simulink subsystem "SimscapePWMModule"  (R2022b)
settings: Solver=VariableStepAuto  StartTime=0.0  StopTime=10.0  RelTol=1e-3
undefined symbols (not defined in the file): DeadTime, fsw
libraries: fl_lib x25
settings Model: Creator=ykamatan  LastModifiedBy=ykamatan

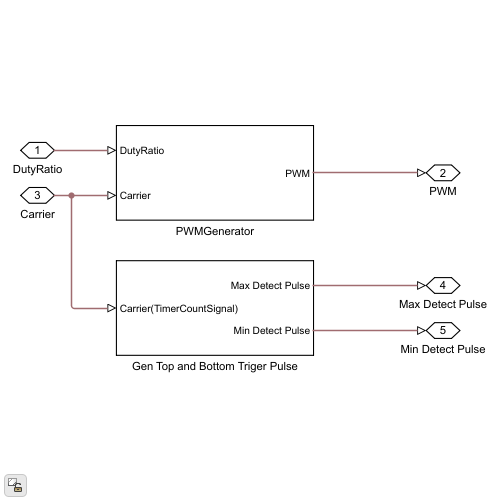
[thumbnail: Simulink's stored preview of the top-level diagram]
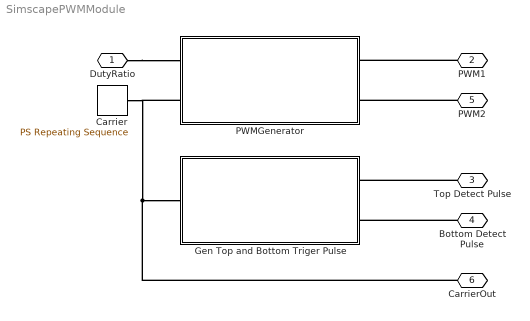
== system SimscapePWMModule ==
  Carrier : fl_lib/Physical Signals/Sources/PS Repeating Sequence  y_init=1  offset=0 s  sig_type=1  durations=[1/fsw/2 1/fsw/2] s  y_start=[1 0]  y_end=[0 1]
      settings: LogSimulationData=on  InternalSimscapePortConfiguration="{\"Bottom\":[],\"Left\":[],\"Right\":[{\"id\":\"Y\",\"label\":\"Y\",\"type\":\"output\"}],\"Top\":[]}"
  Gen Top and Bottom Triger Pulse : Subsystem
  PWMGenerator : Subsystem
  DutyRatio : PMIOPort  Side=Left
  PWM1 : PMIOPort  Port=2  Side=Right
  Top Detect Pulse : PMIOPort  Port=3  Side=Right
  Bottom Detect Pulse : PMIOPort  Port=4  Side=Right
  PWM2 : PMIOPort  Port=5  Side=Right
  CarrierOut : PMIOPort  Port=6  Side=Right
  connections:
  CarrierOut/RConn1 -- Carrier/RConn1 -- PWMGenerator/LConn2 -- Gen Top and Bottom Triger Pulse/LConn1
  Top Detect Pulse/RConn1 -- Gen Top and Bottom Triger Pulse/RConn1
  DutyRatio/RConn1 -- PWMGenerator/LConn1
  Bottom Detect Pulse/RConn1 -- Gen Top and Bottom Triger Pulse/RConn2
  PWM1/RConn1 -- PWMGenerator/RConn1
  PWM2/RConn1 -- PWMGenerator/RConn2

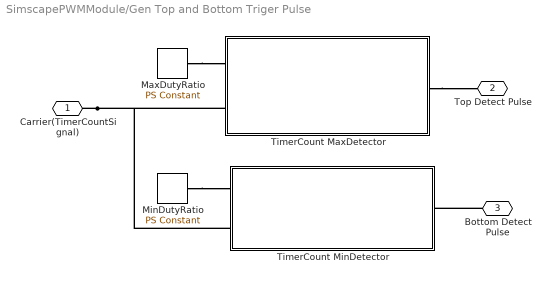
== system SimscapePWMModule/Gen Top and Bottom Triger Pulse ==
  MaxDutyRatio : fl_lib/Physical Signals/Sources/PS Constant  constant=MaxDuty
  MinDutyRatio : fl_lib/Physical Signals/Sources/PS Constant  constant=MinDuty
  TimerCount MaxDetector : Subsystem
  TimerCount MinDetector : Subsystem
  Carrier(TimerCountSignal) : PMIOPort  Side=Left
  Top Detect Pulse : PMIOPort  Port=2  Side=Right
  Bottom Detect Pulse : PMIOPort  Port=3  Side=Right
  connections:
  MaxDutyRatio/RConn1 -- TimerCount MaxDetector/LConn1
  Bottom Detect Pulse/RConn1 -- TimerCount MinDetector/RConn1
  TimerCount MaxDetector/RConn1 -- Top Detect Pulse/RConn1
  MinDutyRatio/RConn1 -- TimerCount MinDetector/LConn1
  Carrier(TimerCountSignal)/RConn1 -- TimerCount MaxDetector/LConn2 -- TimerCount MinDetector/LConn2

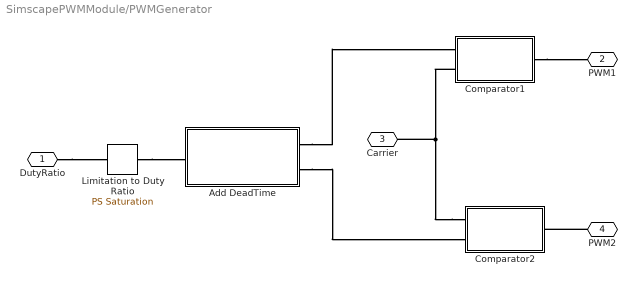
== system SimscapePWMModule/PWMGenerator ==
  Add DeadTime : Subsystem
  Comparator1 : Subsystem
  Comparator2 : Subsystem
  Limitation to Duty Ratio : fl_lib/Physical Signals/Nonlinear Operators/PS Saturation  upper_limit=MaxDuty  lower_limit=MinDuty
  DutyRatio : PMIOPort  Side=Left
  PWM1 : PMIOPort  Port=2  Side=Right
  Carrier : PMIOPort  Port=3  Side=Left
  PWM2 : PMIOPort  Port=4  Side=Right
  connections:
  Comparator1/RConn1 -- PWM1/RConn1
  Add DeadTime/RConn1 -- Comparator1/LConn1
  Comparator2/LConn1 -- Carrier/RConn1 -- Comparator1/LConn2
  Limitation to Duty Ratio/RConn1 -- Add DeadTime/LConn1
  Add DeadTime/RConn2 -- Comparator2/LConn2
  DutyRatio/RConn1 -- Limitation to Duty Ratio/LConn1
  PWM2/RConn1 -- Comparator2/RConn1

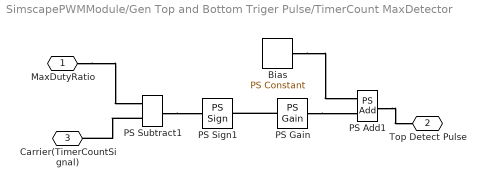
== system SimscapePWMModule/Gen Top and Bottom Triger Pulse/TimerCount MaxDetector ==
  Bias : fl_lib/Physical Signals/Sources/PS Constant  constant=0.5
  PS Add1 : fl_lib/Physical Signals/Functions/PS Add
  PS Gain : fl_lib/Physical Signals/Functions/PS Gain  gain=-0.5
  PS Sign1 : fl_lib/Physical Signals/Nonlinear Operators/PS Sign
      settings: InternalSimscapePortConfiguration="{\"Bottom\":[],\"Left\":[{\"id\":\"I\",\"label\":\"\",\"type\":\"input\"}],\"Right\":[{\"id\":\"O\",\"label\":\"\",\"type\":\"output\"}],\"Top\":[]}"
  PS Subtract1 : fl_lib/Physical Signals/Functions/PS Subtract
  MaxDutyRatio : PMIOPort  Side=Left
  Top Detect Pulse : PMIOPort  Port=2  Side=Right
  Carrier(TimerCountSignal) : PMIOPort  Port=3  Side=Left
  connections:
  PS Add1/RConn1 -- Top Detect Pulse/RConn1
  Bias/RConn1 -- PS Add1/LConn1
  PS Gain/LConn1 -- PS Sign1/RConn1
  PS Gain/RConn1 -- PS Add1/LConn2
  PS Subtract1/LConn2 -- Carrier(TimerCountSignal)/RConn1
  MaxDutyRatio/RConn1 -- PS Subtract1/LConn1
  PS Subtract1/RConn1 -- PS Sign1/LConn1

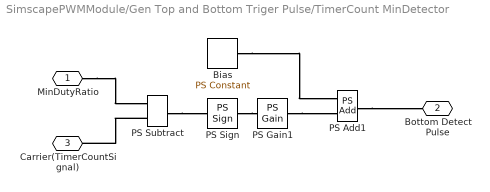
== system SimscapePWMModule/Gen Top and Bottom Triger Pulse/TimerCount MinDetector ==
  Bias : fl_lib/Physical Signals/Sources/PS Constant  constant=0.5
  PS Add1 : fl_lib/Physical Signals/Functions/PS Add
  PS Gain1 : fl_lib/Physical Signals/Functions/PS Gain  gain=0.5
  PS Sign : fl_lib/Physical Signals/Nonlinear Operators/PS Sign
      settings: InternalSimscapePortConfiguration="{\"Bottom\":[],\"Left\":[{\"id\":\"I\",\"label\":\"\",\"type\":\"input\"}],\"Right\":[{\"id\":\"O\",\"label\":\"\",\"type\":\"output\"}],\"Top\":[]}"
  PS Subtract : fl_lib/Physical Signals/Functions/PS Subtract
  MinDutyRatio : PMIOPort  Side=Left
  Bottom Detect Pulse : PMIOPort  Port=2  Side=Right
  Carrier(TimerCountSignal) : PMIOPort  Port=3  Side=Left
  connections:
  PS Gain1/RConn1 -- PS Add1/LConn2
  Bias/RConn1 -- PS Add1/LConn1
  PS Sign/RConn1 -- PS Gain1/LConn1
  PS Subtract/LConn2 -- Carrier(TimerCountSignal)/RConn1
  PS Add1/RConn1 -- Bottom Detect Pulse/RConn1
  PS Subtract/RConn1 -- PS Sign/LConn1
  MinDutyRatio/RConn1 -- PS Subtract/LConn1

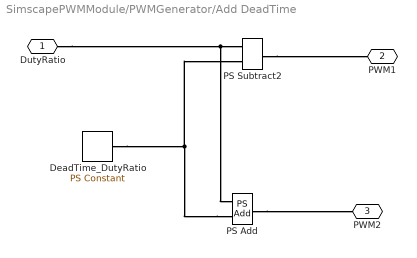
== system SimscapePWMModule/PWMGenerator/Add DeadTime ==
  DeadTime_DutyRatio : fl_lib/Physical Signals/Sources/PS Constant  constant=DeadTime/2*fsw
  PS Add : fl_lib/Physical Signals/Functions/PS Add
  PS Subtract2 : fl_lib/Physical Signals/Functions/PS Subtract
  DutyRatio : PMIOPort  Side=Left
  PWM1 : PMIOPort  Port=2  Side=Right
  PWM2 : PMIOPort  Port=3  Side=Right
  connections:
  PS Add/RConn1 -- PWM2/RConn1
  PS Subtract2/RConn1 -- PWM1/RConn1
  PS Add/LConn2 -- PS Subtract2/LConn2 -- DeadTime_DutyRatio/RConn1
  DutyRatio/RConn1 -- PS Add/LConn1 -- PS Subtract2/LConn1

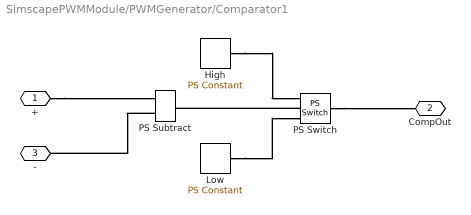
== system SimscapePWMModule/PWMGenerator/Comparator1 ==
  High : fl_lib/Physical Signals/Sources/PS Constant  constant=1
  Low : fl_lib/Physical Signals/Sources/PS Constant  constant=0
  PS Subtract : fl_lib/Physical Signals/Functions/PS Subtract
  PS Switch : fl_lib/Physical Signals/Nonlinear Operators/PS Switch  Threshold=0
      settings: InternalSimscapePortConfiguration="{\"Bottom\":[],\"Left\":[{\"id\":\"I1\",\"label\":\"\",\"type\":\"input\"},{\"id\":\"I2\",\"label\":\"\",\"type\":\"input\"},{\"id\":\"I3\",\"label\":\"\",\"type\":\"input\"}],\"Right\":[{\"id\":\"O\",\"label\":\"\",\"type\":\"output\"}],\"Top\":[]}"
  + : PMIOPort  Side=Left
  CompOut : PMIOPort  Port=2  Side=Right
  - : PMIOPort  Port=3  Side=Left
  connections:
  PS Subtract/LConn2 -- -/RConn1
  PS Switch/RConn1 -- CompOut/RConn1
  High/RConn1 -- PS Switch/LConn1
  +/RConn1 -- PS Subtract/LConn1
  Low/RConn1 -- PS Switch/LConn3
  PS Switch/LConn2 -- PS Subtract/RConn1

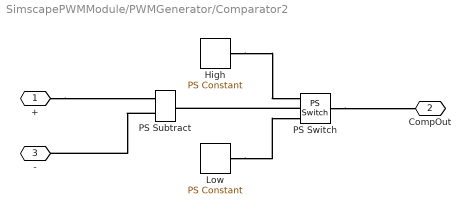
== system SimscapePWMModule/PWMGenerator/Comparator2 ==
  High : fl_lib/Physical Signals/Sources/PS Constant  constant=1
  Low : fl_lib/Physical Signals/Sources/PS Constant  constant=0
  PS Subtract : fl_lib/Physical Signals/Functions/PS Subtract
  PS Switch : fl_lib/Physical Signals/Nonlinear Operators/PS Switch  Threshold=0
      settings: InternalSimscapePortConfiguration="{\"Bottom\":[],\"Left\":[{\"id\":\"I1\",\"label\":\"\",\"type\":\"input\"},{\"id\":\"I2\",\"label\":\"\",\"type\":\"input\"},{\"id\":\"I3\",\"label\":\"\",\"type\":\"input\"}],\"Right\":[{\"id\":\"O\",\"label\":\"\",\"type\":\"output\"}],\"Top\":[]}"
  + : PMIOPort  Side=Left
  CompOut : PMIOPort  Port=2  Side=Right
  - : PMIOPort  Port=3  Side=Left
  connections:
  PS Subtract/LConn2 -- -/RConn1
  PS Switch/RConn1 -- CompOut/RConn1
  High/RConn1 -- PS Switch/LConn1
  +/RConn1 -- PS Subtract/LConn1
  Low/RConn1 -- PS Switch/LConn3
  PS Switch/LConn2 -- PS Subtract/RConn1
